simulink model "hw6"  (R2016b)
settings: Solver=VariableStepAuto  StartTime=0.0  StopTime=10.0  RelTol=1e-3
libraries: elec_lib x14, fl_lib x6
settings Model: Creator=jacob  LastModifiedBy=jacob

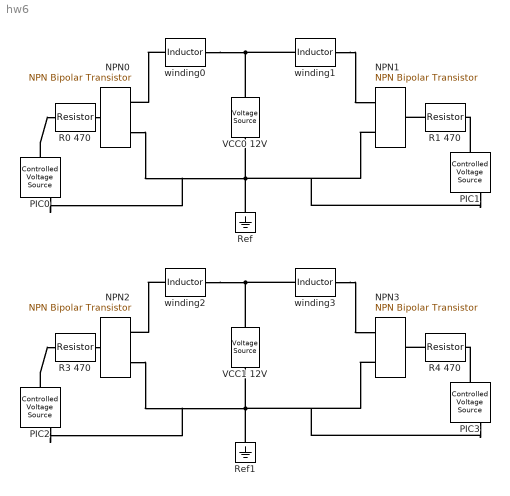
== system hw6 ==
  NPN{0..3} (4 alike) : elec_lib/Semiconductor Devices/NPN Bipolar Transistor  parameterization=1  prmDatasheet=1  prmEquCoeff=1  BF=100  IS=1e-14 A  ec=1  VAF=200 V  hfe=1000  hoe=5e-5 1/Ohm  Ic_h=1 A  Vce_h=4 V  V1=0.7 V  I1=50 mA  BR=1  Tmeas=25 degC  RC=1.5 Ohm  RE=1e-4 Ohm  RB=1 Ohm  C_BC=5 pF  C_BE=5 pF  TF=0 us  TR=0 us  hfe_T2=125  XTB=0  V1_T2=0.45 V  I1_T2=0.5 mA  Tmeas2=125 degC  EG=1.11 eV  XTI=3  TdeviceDatasheet=25 degC  TdeviceEquCoeff=25 degC  Rth=[ 0 10 ] K/W  thermal_mass_parameterization=1  thermal_mass=[ 0 1 ] J/K  thermal_time_constant=[ 0 10 ] s  thermal_mass_initial_temperatures=[ 25 25 ] degC
  PIC{0..3} (4 alike) : fl_lib/Electrical/Electrical Sources/Controlled Voltage Source
  R0 470 : elec_lib/Passive Devices/Resistor  R=470 Ohm  R_tol=5  enable_R_tol=0  tol_distribution=1  nSigma=4  enable_operating_limits=0  operating_limit_action=2  max_working_voltage=100 V  power_rating=1 W  enable_faults=0  fault_action=1  R_faulted=Inf Ohm  enable_temporal_fault=0  t_fault=1 s  enable_behavioral_fault=0  max_permissible_current=1 A  t_fail_on_current=1 s  noise_mode=0  sample_time=0.001 s  repeatability=1  auto_seed=2033606855  user_seed=0  Tdevice=25 degC  alpha=0.00393 1/K  Tmeas=25 degC  thermal_mass=100 J/K  initial_temperature=25 degC  power_derating_T1=70 degC  power_derating_T2=155 degC  operating_temperature_range_vec=[ -50 150 ] degC
  R1 470 : elec_lib/Passive Devices/Resistor  R=470 Ohm  R_tol=5  enable_R_tol=0  tol_distribution=1  nSigma=4  enable_operating_limits=0  operating_limit_action=2  max_working_voltage=100 V  power_rating=1 W  enable_faults=0  fault_action=1  R_faulted=Inf Ohm  enable_temporal_fault=0  t_fault=1 s  enable_behavioral_fault=0  max_permissible_current=1 A  t_fail_on_current=1 s  noise_mode=0  sample_time=0.001 s  repeatability=1  auto_seed=596460160  user_seed=0  Tdevice=25 degC  alpha=0.00393 1/K  Tmeas=25 degC  thermal_mass=100 J/K  initial_temperature=25 degC  power_derating_T1=70 degC  power_derating_T2=155 degC  operating_temperature_range_vec=[ -50 150 ] degC
  R3 470 : elec_lib/Passive Devices/Resistor  R=470 Ohm  R_tol=5  enable_R_tol=0  tol_distribution=1  nSigma=4  enable_operating_limits=0  operating_limit_action=2  max_working_voltage=100 V  power_rating=1 W  enable_faults=0  fault_action=1  R_faulted=Inf Ohm  enable_temporal_fault=0  t_fault=1 s  enable_behavioral_fault=0  max_permissible_current=1 A  t_fail_on_current=1 s  noise_mode=0  sample_time=0.001 s  repeatability=1  auto_seed=1406882827  user_seed=0  Tdevice=25 degC  alpha=0.00393 1/K  Tmeas=25 degC  thermal_mass=100 J/K  initial_temperature=25 degC  power_derating_T1=70 degC  power_derating_T2=155 degC  operating_temperature_range_vec=[ -50 150 ] degC
  R4 470 : elec_lib/Passive Devices/Resistor  R=470 Ohm  R_tol=5  enable_R_tol=0  tol_distribution=1  nSigma=4  enable_operating_limits=0  operating_limit_action=2  max_working_voltage=100 V  power_rating=1 W  enable_faults=0  fault_action=1  R_faulted=Inf Ohm  enable_temporal_fault=0  t_fault=1 s  enable_behavioral_fault=0  max_permissible_current=1 A  t_fail_on_current=1 s  noise_mode=0  sample_time=0.001 s  repeatability=1  auto_seed=2883058518  user_seed=0  Tdevice=25 degC  alpha=0.00393 1/K  Tmeas=25 degC  thermal_mass=100 J/K  initial_temperature=25 degC  power_derating_T1=70 degC  power_derating_T2=155 degC  operating_temperature_range_vec=[ -50 150 ] degC
  Ref : fl_lib/Electrical/Electrical Elements/Electrical Reference
  Ref1 : fl_lib/Electrical/Electrical Elements/Electrical Reference
  VCC0 12V : elec_lib/Sources/Voltage Source  dc_voltage=12 V  ac_voltage=0 V  ac_shift=0 deg  ac_frequency=60 Hz  noise_mode=0  PSD=0 V^2/Hz  sample_time=0.001 s  repeatability=1  auto_seed=1578128389  user_seed=0
  VCC1 12V : elec_lib/Sources/Voltage Source  dc_voltage=12 V  ac_voltage=0 V  ac_shift=0 deg  ac_frequency=60 Hz  noise_mode=0  PSD=0 V^2/Hz  sample_time=0.001 s  repeatability=1  auto_seed=4077229255  user_seed=0
  winding{0..3} (4 alike) : elec_lib/Passive Devices/Inductor  l=10 mH  L_tol=20  enable_L_tol=0  tol_distribution=1  nSigma=4  r=6.2 Ohm  g=1e-9 1/Ohm  initI=0 A  enable_operating_limits=0  operating_limit_action=2  max_working_current=1 A  power_rating=1 W  enable_faults=0  fault_action=1  lambdaPercent=50  k_faulted=0.9999 Ohm  turnsShort=0  openCct=0  groundShort=0  groundShortG=0 1/Ohm  tau_fault=0.001 s  enable_temporal_fault=0  t_fault=1 s  enable_behavioral_fault=0  max_permissible_voltage=100 V  n_fail_on_voltage=1  max_permissible_current=1 A  t_fail_on_current=1 s
  connections:
  VCC0 12V/LConn1 -- winding1/LConn1 -- winding0/RConn1
  Ref/LConn1 -- PIC0/RConn2 -- NPN0/RConn2 -- PIC1/RConn2 -- NPN1/RConn2 -- VCC0 12V/RConn1
  winding0/LConn1 -- NPN0/RConn1
  winding1/RConn1 -- NPN1/RConn1
  R0 470/RConn1 -- NPN0/LConn1
  R1 470/LConn1 -- NPN1/LConn1
  PIC0/LConn1 -- R0 470/LConn1
  PIC1/LConn1 -- R1 470/RConn1
  VCC1 12V/LConn1 -- winding3/LConn1 -- winding2/RConn1
  Ref1/LConn1 -- PIC2/RConn2 -- NPN2/RConn2 -- PIC3/RConn2 -- NPN3/RConn2 -- VCC1 12V/RConn1
  PIC3/LConn1 -- R4 470/RConn1
  winding2/LConn1 -- NPN2/RConn1
  winding3/RConn1 -- NPN3/RConn1
  PIC2/LConn1 -- R3 470/LConn1
  R3 470/RConn1 -- NPN2/LConn1
  R4 470/LConn1 -- NPN3/LConn1
